simulink model "swingup_MPC_controller"  (R2021b)
settings: Solver=FixedStepDiscrete  StartTime=0.0  StopTime=300  FixedStep=h  RelTol=1e-3  EnableMultiTasking=on
PreLoadFcn:
  | warning('off','MATLAB:dispatcher:InexactMatch');
InitFcn:
  | hwinit
values from neighbouring files (symbols this model uses):
  System = c2d(sys_cont, h, 'zoh')    [swingup_mpc_init.m]
undefined symbols (not defined in the file or in its folder): Discrete, MPCparams, Time
libraries: simulink x1, ctrlSharedLib x1, embmathops x1
settings Model: SimulationMode=external  ExtModeTrigDuration=100000  Creator=user  LastModifiedBy=liamligthart
settings SolverCC: AlgebraicLoopSolver=TrustRegion
settings DataIOCC: SaveFormat=Array  SignalLoggingSaveFormat=ModelDataLogs  SaveOutput=off  SignalLogging=off  DSMLogging=off  SaveTime=off  ReturnWorkspaceOutputs=off
settings OptimizationCC: ExpressionDepthLimit=2147483647  LifeSpan=inf
settings DebuggingCC: MergeDetectMultiDrivingBlocksExec=none  SolverPrmCheckMsg=warning  FcnCallInpInsideContextMsg=warning  StateNameClashWarn=warning  SFUnexpectedBacktrackingDiag=warning  SFNoUnconditionalDefaultTransitionDiag=warning  SFExecutionAtInitializationDiag=none  SFMachineParentedDataDiag=warning  ArithmeticOperatorsInVariantConditions=warning
settings HardwareCC: ProdBitPerPointer=32  ProdBitPerSizeT=32  ProdBitPerPtrDiffT=32  ProdLargestAtomicFloat=None  ProdIntDivRoundTo=Undefined  ProdEndianess=Unspecified  ProdWordSize=32  ProdHWDeviceType=32-bit Generic
settings ModelReferenceCC: PropagateSignalLabelsOutOfModel=off
settings SFSimCC: SimUseLocalCustomCode=off  CustomCodeUndefinedFunction=UseInterfaceOnly
settings RTWCC: Description=rpend RTDAC/USB2 (Visual C/C++)  SystemTargetFile=rtcon_rpend_usb2.tlc  TemplateMakefile=rtcon_rpend_vc_usb2_x64.tmf  RTWUseLocalCustomCode=off
settings CodeAppCC: StateflowObjectComments=on
settings STFCustomTargetCC: ModelReferenceCompliant=off  CombineOutputUpdateFcns=on  MatFileLogging=on  GRTInterface=off  SystemTargetFile=rtcon_rpend_usb2.tlc
settings GRTTargetCC: TargetLangStandard=C89/C90 (ANSI)  ModelReferenceCompliant=off  ParMdlRefBuildCompliant=off  CompOptLevelCompliant=off  ConcurrentExecutionCompliant=off  CPPClassGenCompliant=off  UseToolchainInfoCompliant=off  ExtMode=on  ExtModeMexFile=rtcon_ext_comm
settings ConfigComp: CovMetricSettings=dw  CovSaveCumulativeToWorkspaceVar=on  CovSaveSingleToWorkspaceVar=on  CovExternalEMLEnable=off  CovSFcnEnable=off

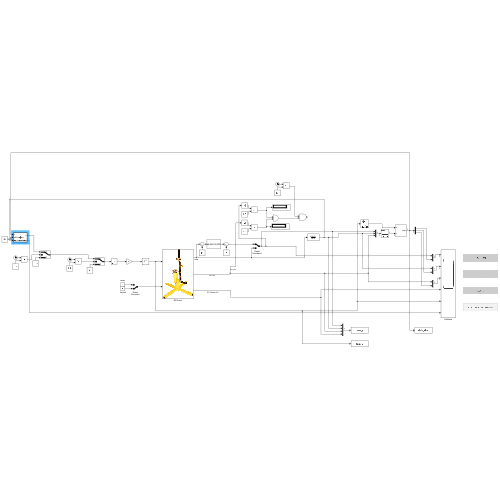
[thumbnail: Simulink's stored preview of the top-level diagram]
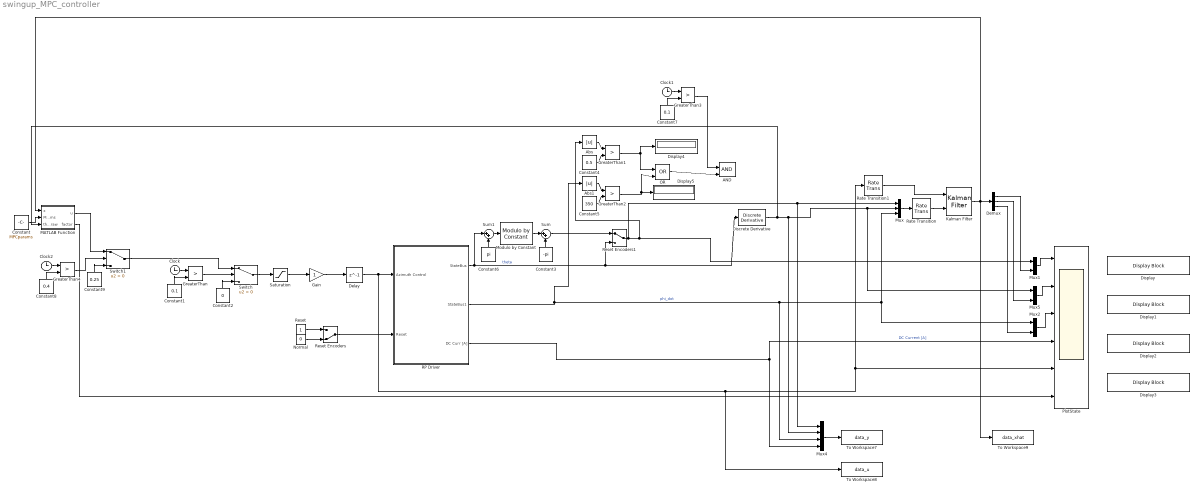
== system swingup_MPC_controller ==
  AND : Logic  IconShape=distinctive  AllPortsSameDT=off  OutDataTypeStr=boolean
  Abs : Abs
  Abs1 : Abs
  Clock : Clock
  Clock1 : Clock
  Clock2 : Clock
  Constant : Constant  Value=MPCparams  VectorParams1D=off  OutDataTypeStr=Bus: MPCparams_bus
  Constant1 : Constant  Value=0.1
  Constant2 : Constant  Value=0
  Constant3 : Constant  Value=-pi
  Constant4 : Constant  Value=0.5
  Constant5 : Constant  Value=350
  Constant6 : Constant  Value=pi
  Constant7 : Constant  Value=0.1
  Constant8 : Constant  Value=0.4
  Constant9 : Constant  Value=0.25
  Delay : Delay  DelayLength=1  InitialCondition=0
  Demux : Demux  Outputs=3
  Discrete Derivative : simulink/Discrete/Discrete Derivative  gainval=1.0  ICPrevScaledInput=0.0  OutMin=[]  OutMax=[]  OutDataType=fixdt(1, 16)  OutScaling=2^-10  DoSatur=off
  Display{,1..3} (4 alike) : DisplayBlock  LabelPosition=Hide  Format=short  Transparency=1
  Display4 : Display
  Display5 : Display
  Gain : Gain
  GreaterThan{,1..4} (5 alike) : RelationalOperator  Priority=0  Operator=>  OutDataTypeStr=boolean  RndMeth=Simplest
  Kalman Filter : ctrlSharedLib/Kalman Filter  TimeDomain=Discrete-Time  UseCurrentEstimator=on  ModelSource=Individual A, B, C, D matrices  ModelSourceVariable=ss(0.95,1,1,0,1)  A=System.A  B=System.B  C=eye(3)  D=zeros(3,1)  NumberOfStates=1  NumberOfInputs=1  NumberOfOutputs=1  InitialEstimateSource=Dialog  X0=[0;0;0]  P0=10  UseK=off  UseGH=off  NumberOfProcessNoiseInputs=1  G=1  TimeInvariantG=on  H=0  TimeInvariantH=on  Q=diag([0.05,0.001,0.1])  TimeInvariantQ=on  R=diag([0.001,0.01,0.01])  TimeInvariantR=on  N=0  TimeInvariantN=on  AddInputPort=on  AddEnablePort=off  OutputEstimatedY=off  OutputP=off  Ts=-1
  MATLAB Function : MATLAB Function  TreatAsAtomicUnit=on
  Modulo by Constant : embmathops/Modulo by Constant  Denominator=2*pi  SimulateUsing=Code generation
      settings: SourceProductBaseCode=SL
  Mux : Mux  Inputs=3
  Mux1 : Mux  Inputs=2
  Mux2 : Mux  Inputs=2
  Mux4 : Mux
  Mux5 : Mux  Inputs=2
  Normal : Constant  Value=0
  OR : Logic  Operator=OR  IconShape=distinctive  AllPortsSameDT=off  OutDataTypeStr=boolean
  PlotState : Scope  NumInputPorts=6
  RP Driver : Subsystem
      mask Display: image(imread('rwp.JPG'))
  Rate Transition : RateTransition  OutPortSampleTime=0.05
  Rate Transition1 : RateTransition  OutPortSampleTime=0.05
  Reset : Constant
  Reset Encoders : ManualSwitch  CurrentSetting=0
  Reset Encoders1 : ManualSwitch
  Saturation : Saturate  UpperLimit=1  LowerLimit=-1
  Sum : Sum  Inputs=|++
  Sum1 : Sum  Inputs=|++
  Switch : Switch  Criteria=u2 > Threshold
  Switch1 : Switch  Criteria=u2 > Threshold
  To Workspace7 : ToWorkspace  VariableName=data_y  SaveFormat=Timeseries  SampleTime=-1
  To Workspace8 : ToWorkspace  VariableName=data_u  SaveFormat=Timeseries  SampleTime=-1
  To Workspace9 : ToWorkspace  VariableName=data_xhat  SaveFormat=Timeseries  SampleTime=-1
  wires:
  Normal/1 -> Reset Encoders/2
  Reset/1 -> Reset Encoders/1
  Reset Encoders/1 -> RP Driver/2(Reset)
  RP Driver/3(DC Curr [A]) -> Mux4/4, PlotState/4  "DC Current [A]"
  RP Driver/2(StateBus1) -> Abs1/1, Mux4/3, Mux/3, Mux2/1  "phi_dot"
  Mux1/1 -> PlotState/1
  Demux/1 -> Mux1/2
  Demux/3 -> Mux2/2
  Mux2/1 -> PlotState/3
  Kalman Filter/1 -> To Workspace9/1, Demux/1, MATLAB Function/1(x)
  Mux/1 -> Rate Transition/1
  Rate Transition/1 -> Kalman Filter/2
  Clock/1 -> GreaterThan/1
  Constant1/1 -> GreaterThan/2
  GreaterThan/1 -> Switch/2
  Constant2/1 -> Switch/3
  Rate Transition1/1 -> Kalman Filter/1
  Delay/1 -> To Workspace8/1, Rate Transition1/1, PlotState/5, RP Driver/1(Azimuth Control)
  Saturation/1 -> Gain/1
  Switch/1 -> Saturation/1
  RP Driver/1(StateBus) -> Sum1/1, Discrete Derivative/1, Reset Encoders1/2  "theta"
  Constant3/1 -> Sum/2
  Modulo by Constant/1 -> Sum/1
  Gain/1 -> Delay/1
  Sum/1 -> Reset Encoders1/1
  Reset Encoders1/1 -> Abs/1, Mux1/1, Mux4/1, Mux/1
  Discrete Derivative/1 -> MATLAB Function/3(th_dot_raw), Mux4/2, Mux5/1, Mux/2
  Abs/1 -> GreaterThan1/1
  Constant4/1 -> GreaterThan1/2
  GreaterThan1/1 -> OR/1, Display4/1
  Constant5/1 -> GreaterThan2/2
  GreaterThan2/1 -> Display5/1, OR/2
  Abs1/1 -> GreaterThan2/1
  Constant/1 -> MATLAB Function/2(MPCparams)
  Mux4/1 -> To Workspace7/1
  Mux5/1 -> PlotState/2
  Demux/2 -> Mux5/2
  Constant6/1 -> Sum1/2
  Sum1/1 -> Modulo by Constant/1
  Constant7/1 -> GreaterThan3/2
  Clock1/1 -> GreaterThan3/1
  GreaterThan3/1 -> AND/1
  OR/1 -> AND/2
  GreaterThan4/1 -> Switch1/2
  Clock2/1 -> GreaterThan4/1
  Constant8/1 -> GreaterThan4/2
  Constant9/1 -> Switch1/3
  MATLAB Function/1(u) -> Switch1/1
  Switch1/1 -> Switch/1
  MATLAB Function/2(factor) -> PlotState/6

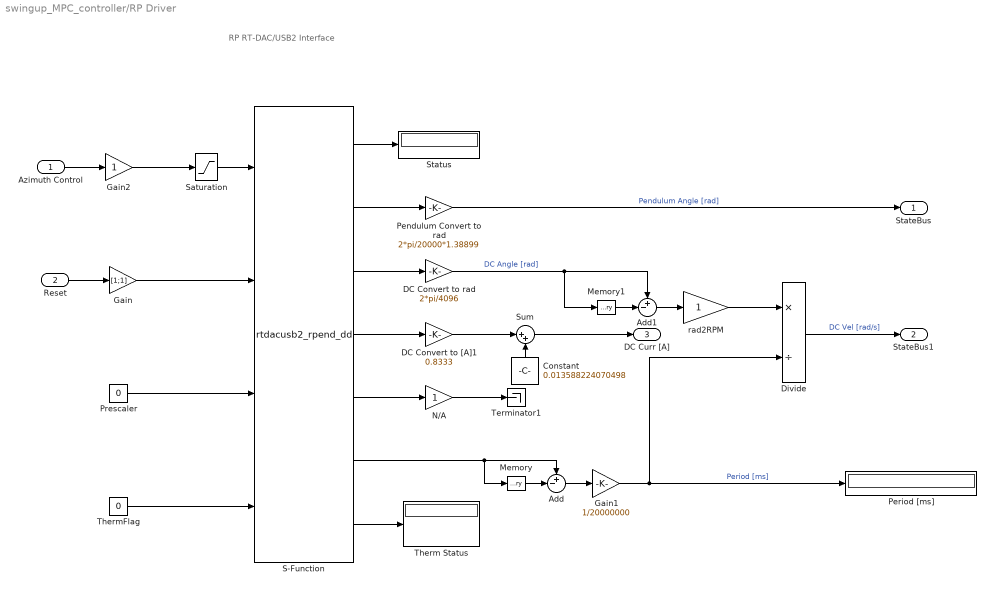
== system swingup_MPC_controller/RP Driver ==
  note: RP RT-DAC/USB2
      | Interface
  Azimuth Control : Inport
  Reset : Inport  Port=2
  Add : Sum  Inputs=+-|
  Add1 : Sum  Inputs=+-|
  Constant : Constant  Value=0.013588224070498
  DC Convert to [A]1 : Gain  Gain=0.8333  SaturateOnIntegerOverflow=on  OutDataTypeStr=Inherit: Same as input  ParamDataTypeStr=Inherit: Same as input
  DC Convert to rad : Gain  Gain=2*pi/4096  SaturateOnIntegerOverflow=on  OutDataTypeStr=Inherit: Same as input  ParamDataTypeStr=Inherit: Same as input
  Divide : Product  Inputs=*/
  Gain : Gain  Gain=[1;1]
  Gain1 : Gain  Gain=1/20000000
  Gain2 : Gain
  Memory : Memory
  Memory1 : Memory
  N/A : Gain  SaturateOnIntegerOverflow=on  OutDataTypeStr=Inherit: Same as input  ParamDataTypeStr=Inherit: Same as input
  Pendulum Convert to rad : Gain  Gain=2*pi/20000*1.38899  SaturateOnIntegerOverflow=on  OutDataTypeStr=Inherit: Same as input  ParamDataTypeStr=Inherit: Same as input
  Period [ms] : Display
  Prescaler : Constant  Value=0
  S-Function : S-Function  FunctionName=rtdacusb2_rpend_dd  Parameters=1, h  SFunctionDeploymentMode=off  EnableBusSupport=off
  Saturation : Saturate  UpperLimit=1  LowerLimit=-1
  Status : Display
  Sum : Sum  Inputs=|++
  Terminator1 : Terminator
  Therm Status : Display
  ThermFlag : Constant  Value=0
  rad2RPM : Gain  SaturateOnIntegerOverflow=on  OutDataTypeStr=Inherit: Same as input  ParamDataTypeStr=Inherit: Same as input
  StateBus : Outport  VectorParamsAs1DForOutWhenUnconnected=off
  StateBus1 : Outport  Port=2  VectorParamsAs1DForOutWhenUnconnected=off
  DC Curr [A] : Outport  Port=3  VectorParamsAs1DForOutWhenUnconnected=off
  wires:
  S-Function/7 -> Therm Status/1
  S-Function/5 -> N/A/1
  S-Function/4 -> DC Convert to [A]1/1
  ThermFlag/1 -> S-Function/4
  Prescaler/1 -> S-Function/3
  Gain/1 -> S-Function/2
  Divide/1 -> StateBus1/1  "DC Vel [rad/s]"
  rad2RPM/1 -> Divide/1
  Add1/1 -> rad2RPM/1
  Memory1/1 -> Add1/2
  N/A/1 -> Terminator1/1
  S-Function/6 -> Add/1, Memory/1
  Gain2/1 -> Saturation/1
  Gain1/1 -> Period [ms]/1, Divide/2  "Period [ms]"
  Add/1 -> Gain1/1
  Memory/1 -> Add/2
  DC Convert to rad/1 -> Add1/1, Memory1/1  "DC Angle [rad]"
  S-Function/3 -> DC Convert to rad/1
  Pendulum Convert to rad/1 -> StateBus/1  "Pendulum Angle [rad]"
  S-Function/2 -> Pendulum Convert to rad/1
  S-Function/1 -> Status/1
  Saturation/1 -> S-Function/1
  Reset/1 -> Gain/1
  Azimuth Control/1 -> Gain2/1
  DC Convert to [A]1/1 -> Sum/1
  Sum/1 -> DC Curr [A]/1
  Constant/1 -> Sum/2

== matlab function swingup_MPC_controller/MATLAB Function ==
  data: x input; u output; MPCparams input; factor output; th_dot_raw input
function [u, factor] = swingup_mpc_controller(x, MPCparams, th_dot_raw)
    % Inputs:
    % x:            observer state at current time [nx x 1]
    % MPCparams:    struct with all offline MPC calculations
    %
    % Outputs:
    % u:            optimal input at current time [1 x 1]
    
    % Initialize u
    factor = 0;
    u = zeros(1,1);


    swingup = 0;
    % Find out if we are within the controllable bounds
    if(abs(x(1)) > 0.4)
        swingup = 1;
    end

    if(swingup == 0)
        % Compute linear part of cost function (dependent on x0)
        f_i = MPCparams.CostMatrices.f * x;
    
        % Compute bound vector on u (dependent on x0)
        b_i = [MPCparams.Bounds.bx - MPCparams.Bounds.Ax * MPCparams.PredMatrices.T * x; MPCparams.Bounds.bu];
        
        % Do the optimization
        %coder.extrinsic('quadprog');
        [u_opt, ~, exitflag, ~] = quadprog(MPCparams.CostMatrices.H, f_i, MPCparams.Bounds.A, b_i, [], [], [], [], zeros(size(f_i)), optimoptions('quadprog', Display='off', Algorithm='active-set'));
    
        if exitflag ~= 1
            disp("WARNING: exitflag = " + exitflag);
            if x(2) > 0
                u = -1;
            else
                u = 1;
            end
        else
            u = u_opt(1);
        end
    end

    % DO SWINGUP IF OUT OF CONTROLLABLE BOUNDS
    if(swingup)
        factor = 1 - (0.5 * 1/MPCparams.Swingup.a4 * th_dot_raw^2 + cos(x(1))) / MPCparams.Swingup.friction_compensation;
        u = -sign(th_dot_raw) * MPCparams.Swingup.max * factor;
    end


 
end
